simulink model "Experiment_1_cs"  (R2022b)
settings: Solver=ode5  StartTime=0.0  StopTime=30  FixedStep=1/20  RelTol=1e-3
PreLoadFcn:
  | mbxruntime.callbacks.PreLoadFcn(bdroot);
PostLoadFcn:
  | mbxruntime.callbacks.PostLoadFcn(bdroot);
InitFcn:
  | mbxruntime.callbacks.InitFcn(bdroot);
StartFcn:
  | mbxruntime.callbacks.StartFcn(bdroot);
StopFcn:
  | mbxruntime.callbacks.StopFcn(bdroot);
model workspace (MAT data in the model file):
  mbox_table : object (value not decoded)
  model_closed = 0
  sim_status = 0
undefined symbols (not defined in the file or in its folder): blockPath, DiscIntNeverNeededParam, warningInitialVelocity, x0
libraries: PreScanSimulinkLibrary x32, simulink x23, simulink_extras x10
(part 7 of 8)

== system Experiment_1_cs/Male_Old_White_WithStick_1/Trajectories/Traj2State1/Traj2State2/Traj2MuxState_Ext/demux ==
  traj : Inport
  Demux : Demux  Outputs=18
  x : Outport
  y : Outport  Port=2
  z : Outport  Port=3
  velx : Outport  Port=4
  vely : Outport  Port=5
  velz : Outport  Port=6
  R : Outport  Port=7
  P : Outport  Port=8
  Y : Outport  Port=9
  velR : Outport  Port=10
  velP : Outport  Port=11
  velY : Outport  Port=12
  accx : Outport  Port=13
  accy : Outport  Port=14
  accz : Outport  Port=15
  accR : Outport  Port=16
  accP : Outport  Port=17
  accY : Outport  Port=18
  wires:
  Demux/18 -> accY/1
  Demux/17 -> accP/1
  Demux/16 -> accR/1
  Demux/15 -> accz/1
  Demux/14 -> accy/1
  Demux/13 -> accx/1
  Demux/12 -> velY/1
  Demux/11 -> velP/1
  Demux/10 -> velR/1
  Demux/9 -> velz/1
  Demux/8 -> vely/1
  Demux/7 -> velx/1
  Demux/6 -> Y/1
  Demux/5 -> P/1
  traj/1 -> Demux/1
  Demux/4 -> R/1
  Demux/3 -> z/1
  Demux/2 -> y/1
  Demux/1 -> x/1

== system Experiment_1_cs/Man_200_1/Trajectories/Traj2State1/Traj2State2/Traj2MuxState_Ext/demux ==
  traj : Inport
  Demux : Demux  Outputs=18
  x : Outport
  y : Outport  Port=2
  z : Outport  Port=3
  velx : Outport  Port=4
  vely : Outport  Port=5
  velz : Outport  Port=6
  R : Outport  Port=7
  P : Outport  Port=8
  Y : Outport  Port=9
  velR : Outport  Port=10
  velP : Outport  Port=11
  velY : Outport  Port=12
  accx : Outport  Port=13
  accy : Outport  Port=14
  accz : Outport  Port=15
  accR : Outport  Port=16
  accP : Outport  Port=17
  accY : Outport  Port=18
  wires:
  Demux/18 -> accY/1
  Demux/17 -> accP/1
  Demux/16 -> accR/1
  Demux/15 -> accz/1
  Demux/14 -> accy/1
  Demux/13 -> accx/1
  Demux/12 -> velY/1
  Demux/11 -> velP/1
  Demux/10 -> velR/1
  Demux/9 -> velz/1
  Demux/8 -> vely/1
  Demux/7 -> velx/1
  Demux/6 -> Y/1
  Demux/5 -> P/1
  traj/1 -> Demux/1
  Demux/4 -> R/1
  Demux/3 -> z/1
  Demux/2 -> y/1
  Demux/1 -> x/1

== system Experiment_1_cs/Nissan_Cabstar_Boxtruck_1/Trajectories/Traj2State1/Traj2State2/Traj2MuxState_Ext/demux ==
  traj : Inport
  Demux : Demux  Outputs=18
  x : Outport
  y : Outport  Port=2
  z : Outport  Port=3
  velx : Outport  Port=4
  vely : Outport  Port=5
  velz : Outport  Port=6
  R : Outport  Port=7
  P : Outport  Port=8
  Y : Outport  Port=9
  velR : Outport  Port=10
  velP : Outport  Port=11
  velY : Outport  Port=12
  accx : Outport  Port=13
  accy : Outport  Port=14
  accz : Outport  Port=15
  accR : Outport  Port=16
  accP : Outport  Port=17
  accY : Outport  Port=18
  wires:
  Demux/18 -> accY/1
  Demux/17 -> accP/1
  Demux/16 -> accR/1
  Demux/15 -> accz/1
  Demux/14 -> accy/1
  Demux/13 -> accx/1
  Demux/12 -> velY/1
  Demux/11 -> velP/1
  Demux/10 -> velR/1
  Demux/9 -> velz/1
  Demux/8 -> vely/1
  Demux/7 -> velx/1
  Demux/6 -> Y/1
  Demux/5 -> P/1
  traj/1 -> Demux/1
  Demux/4 -> R/1
  Demux/3 -> z/1
  Demux/2 -> y/1
  Demux/1 -> x/1

== system Experiment_1_cs/Audi_A8_Sedan_1/Dynamics_Simple/Chassis/Bicycle_model_[XYZ]/X_Motion/Max RPM and zero- velocity detection/Configurable Subsystem ==
  Step : Step  Time=0.0001  Before=1  After=0  SampleTime=0
  Out1 : Outport
  wires:
  Step/1 -> Out1/1

== system Experiment_1_cs/Audi_A8_Sedan_1/Dynamics_Simple/Chassis/Bicycle_model_[XYZ]/X_Motion/Max RPM and zero- velocity detection/SR-Memory ==
  Signal : Inport
  Set : Inport  Port=2
  Reset : Inport  Port=3
  Constant : Constant  Value=0
  Detect Rise Positive : simulink/Logic and Bit Operations/Detect Rise Positive  vinit=0  OutDataTypeStr=uint8
  Detect Rise Positive1 : simulink/Logic and Bit Operations/Detect Rise Positive  vinit=0  OutDataTypeStr=uint8
  Manual Switch : ManualSwitch
  Manual Switch1 : ManualSwitch
  Switch : Switch  Criteria=u2 ~= 0  SaturateOnIntegerOverflow=off  InputSameDT=off
  Switch1 : Switch  Criteria=u2 ~= 0  SaturateOnIntegerOverflow=off  InputSameDT=off
  Unit Delay : UnitDelay  SampleTime=-1  HasFrameUpgradeWarning=on
  Out : Outport
  wires:
  Constant/1 -> Switch1/1
  Switch/1 -> Switch1/3
  Switch1/1 -> Unit Delay/1, Out/1
  Manual Switch1/1 -> Switch1/2
  Reset/1 -> Manual Switch1/2, Detect Rise Positive1/1
  Detect Rise Positive1/1 -> Manual Switch1/1
  Signal/1 -> Switch/1
  Unit Delay/1 -> Switch/3
  Set/1 -> Detect Rise Positive/1, Manual Switch/2
  Detect Rise Positive/1 -> Manual Switch/1
  Manual Switch/1 -> Switch/2

== matlab function Experiment_1_cs/Audi_A8_Sedan_1/perception module/MATLAB Function2 ==
  data: obs_x input; obs_y input; obs_v input; obs_heading input; obs_id input
function plot_obstacles_vcs(obs_x, obs_y, obs_v, obs_heading, obs_id)
% Simulink-friendly Visualization Function

% 声明绘图函数为 extrinsic
coder.extrinsic('figure','clf','hold','grid','axis','xlim','ylim','xlabel','ylabel','title');
coder.extrinsic('plot','quiver','text','fill','legend');
coder.extrinsic('sprintf');

persistent figCreated;

% 初始化图
if isempty(figCreated)
    figure(100);
    figCreated = true;
end

figure(100);
clf; hold on; grid on; axis equal;

% 坐标范围
xlim([-20 80]);
ylim([-50 50]);
xlabel('X_{VCS} (m)');
ylabel('Y_{VCS} (m)');
title('Obstacle Positions in VCS');

%% ======================
%       主车矩形
% ======================
Lh = 5;   % 主车长
Wh = 2;   % 主车宽
hd = 0;   % 主车朝向始终沿 +X

% 主车矩形点
rect_host = [
    Lh/2,  Wh/2;
    Lh/2, -Wh/2;
   -Lh/2, -Wh/2;
   -Lh/2,  Wh/2
];

% 主车旋转矩阵
R = [cos(hd) -sin(hd); sin(hd) cos(hd)];
rect_host_rot = (R * rect_host')';
rect_host_final = rect_host_rot + [0, 0];

% 绘制主车矩形（蓝色）
fill(rect_host_final(:,1), rect_host_final(:,2), ...
    [0.2 0.6 1.0], 'FaceAlpha',0.4, 'EdgeColor','b', 'LineWidth',2);

text(0, -1.5, 'Host Car', 'Color','b','FontSize',12,'FontWeight','bold');

%% ======================
%       障碍物绘制
% ======================
for i = 1:length(obs_x)
    if isnan(obs_x(i)), continue; end

    ox = obs_x(i);
    oy = obs_y(i);
    v  = obs_v(i);
    hd = obs_heading(i);
    oid = obs_id(i);

    % 速度箭头
    quiver(ox, oy, v*cos(hd), v*sin(hd), 0.5, 'b', 'LineWidth', 1.5);

    %% ========== 障碍车辆 (ID == 42/54) ==========
    if oid == 42 || oid == 54
        L = 5; W = 2;

        rect = [
            L/2,  W/2;
            L/2, -W/2;
           -L/2, -W/2;
           -L/2,  W/2
        ];

        R = [cos(hd) -sin(hd); sin(hd) cos(hd)];
        rect_rot = (R * rect')';
        rect_final = rect_rot + [ox, oy];

        fill(rect_final(:,1), rect_final(:,2), [0.3 0.8 0.3], ...
            'FaceAlpha',0.4, 'EdgeColor','g', 'LineWidth',2);

        text(ox, oy, 'Car(42)', 'Color','g','FontSize',12,'FontWeight','bold');

    else
        %% 普通障碍物
        plot(ox, oy, 'ro', 'MarkerFaceColor', 'r');
        text(ox + 0.3, oy + 0.3, sprintf('%d', int32(oid)), ...
            'Color','y','FontSize',12,'FontWeight','bold');
    end
end

legend('Velocity','Host');

end

== matlab function Experiment_1_cs/Cloud Computing Systerm/Dangerous Check/MATLAB Function ==
  settings: updateMethod=DISCRETE
  data: no_signal_zone_x input; ego_y input; lane0_y input; target_y output; lane1_y input; lane2_y input; last_target_y input; obs_x_set_gcs input; obs_y_set_gcs input; obs_v_set_gcs input; obs_heading_set_gcs input; obs_ID_set input; ego_x input; ego_v input; ego_heading input; ego_yawrate input; last_target_v input; target_v output; time input; out_state output; has_signal output; danger_level output; action output; collision_info output Bus: collision_info_bus
function [target_y, target_v, out_state, has_signal, danger_level, action, collision_info] = ...
    fcn(no_signal_zone_x, ego_y, lane0_y, lane1_y, lane2_y, last_target_y, ...
        obs_x_set_gcs, obs_y_set_gcs, obs_v_set_gcs, obs_heading_set_gcs, ...
        obs_ID_set, ego_x, ego_v, ego_heading, ego_yawrate, last_target_v, time)


%% ------------------------------------------------------
% Persistent Variables
%% ------------------------------------------------------
persistent first_run stored_target_y stored_target_v state block_until_time
action = 0;
collision_info.obs_id = int32(-1);
collision_info.time = -1;

if isempty(first_run)
    first_run = true;
    stored_target_y = 0;
    stored_target_v = 0;
    state = 0;
    block_until_time = 0;
end

%% Parameters
dt = 0.05;
recommond_speed = 15;
lane_width = 3.5;
max_acc = 2;
max_de_acc = -3.5;

ego_heading = wrapToPi(-deg2rad(ego_heading - 90));
lane_y_all = [lane0_y, lane1_y, lane2_y];

%% Signal availability
has_signal = (ego_x < no_signal_zone_x);

%% =============== CASE 1: LOST SIGNAL ===================
if ~has_signal
    stored_target_v = 0;
    stored_target_y = 0;
    state = 0;

    % Danger level 依旧保留
    danger_level = calc_lost_signal_danger( ...
        ego_x, ego_y, ego_heading, ...
        obs_x_set_gcs, obs_y_set_gcs, obs_v_set_gcs, obs_heading_set_gcs, ...
        obs_ID_set, lane_y_all, lane_width);

    % ⭐ 新增：调用 analyze_danger
    [danger_ns, tx_ns] = analyze_danger( ...
        ego_x, ego_y, ego_v, ego_heading, ...
        obs_x_set_gcs, obs_y_set_gcs, obs_v_set_gcs, ...
        obs_heading_set_gcs, obs_ID_set, lane_y_all, lane_width);

    % 找最危险 lane（TTC 最小）
    ttc_list = tx_ns(:,1);
    [min_ttc, idx_lane] = min(ttc_list);

    if min_ttc < 99
        collision_info.obs_id = int32(danger_ns(idx_lane,2));
        collision_info.time   = min_ttc;
    else
        collision_info.obs_id = int32(-1);
        collision_info.time   = 999;
    end

    % 输出保持
    target_v = stored_target_v;
    target_y = stored_target_y;
    out_state = state;
    action = 0;
    return;
end

%% =============== FIRST RUN ===================
if first_run
    [~, idx_lane] = min(abs(ego_y - lane_y_all));
    stored_target_y = lane_y_all(idx_lane);
    stored_target_v = recommond_speed;

    first_run = false;

    target_y = stored_target_y;
    target_v = stored_target_v;
    out_state = state;
    danger_level = 0;
    action = 0;
    return;
end

%% =============== NORMAL MODE ===================
stored_target_y = last_target_y;
stored_target_v = last_target_v;

%% Danger Analysis
[danger, tx_lane] = analyze_danger( ...
    ego_x, ego_y, ego_v, ego_heading, ...
    obs_x_set_gcs, obs_y_set_gcs, obs_v_set_gcs, obs_heading_set_gcs, obs_ID_set, ...
    lane_y_all, lane_width);

% Determine lane index (scalar)
lane_idx = 1;
min_val = abs(stored_target_y - lane_y_all(1));
for ii = 2:3
    if abs(stored_target_y - lane_y_all(ii)) < min_val
        min_val = abs(stored_target_y - lane_y_all(ii));
        lane_idx = ii;
    end
end

is_danger = danger(lane_idx, 1);
t_lane  = tx_lane(lane_idx, 1);
x_lane  = tx_lane(lane_idx, 2);
if is_danger
    collision_info.obs_id = int32(danger(lane_idx, 2));
    collision_info.time = t_lane;
end

%% --------------------- State Machine ---------------------
switch state

case 0   % KEEP
    action = 0;
    block_until_time = time;

    if is_danger
        state = 1;
    else
        stored_target_v = min(stored_target_v + max_acc*dt, recommond_speed);
    end

case 1   % BRAKE
    if is_danger
        d_brake = ego_v^2 / (2*abs(max_de_acc));
        dx_conflict = x_lane - ego_x;

        if d_brake < dx_conflict - 6
            stored_target_v = last_target_v + max_de_acc * dt;
            action = 2;

            obs_id = danger(lane_idx,2);
            idx_obs = find(obs_ID_set == obs_id, 1);
            if isempty(idx_obs), idx_obs = 1; end

            vy = obs_v_set_gcs(idx_obs) * sin(obs_heading_set_gcs(idx_obs));

            block_until_time = time + min(t_lane, (lane_width/2)/max(abs(vy),0.01));

        else
            % change lane
            
            if lane_idx == 1
                cand = 2;
            elseif lane_idx == 3
                cand = 2;
            else
                cand = [1, 3];
            end
        
            % 从候选车道里找一个安全车道
            new_lane = lane_idx; % 默认保持
            for ci = 1:length(cand)
                if ~danger(cand(ci),1)
                    new_lane = cand(ci);
                    break;
                end
            end

            stored_target_y = lane_y_all(new_lane);
            state = 2;
            action = 3;
        end

        % failsafe: too slow but still dangerous
        obs_id = danger(lane_idx, 2);
        obs_v_risk = 999;
        % 手写一个确定的标量查找
        for ii = 1:length(obs_ID_set)
            if obs_ID_set(ii) == obs_id
                obs_v_risk = obs_v_set_gcs(ii);
                break;
            end
        end
        if (ego_v < 5 || obs_v_risk < 0.2)&& is_danger
            new_lane = lane_idx;
            found = false;

            for li = 1:3
                if danger(li,1)==false
                    new_lane = li;
                    found = true;
                    break;
                end
            end

            if ~found
                action = 4;
            else
                stored_target_y = lane_y_all(new_lane);
                state = 2;
            end
        end

    else
        state = 3;
        action = 1;
    end

case 2   % CHANGE LANE
    block_until_time = time + 0.5;
    stored_target_v = last_target_v;
    state = 3;
    action = 3;

case 3   % BLOCK
    if time >= block_until_time
        state = 0;
    end
    stored_target_v = last_target_v;
    action = 1;

end

%% Outputs
target_y = stored_target_y;
target_v = stored_target_v;
out_state = state;
danger_level = 0;

end  % END fcn


%% =====================================================================
%%                        analyze_danger
%% =====================================================================
function [danger, tx_lane] = analyze_danger( ...
    ego_x, ego_y, ego_v, ego_heading, ...
    obs_x, obs_y, obs_v, obs_h, obs_ID, lane_y, lane_width)

N = length(obs_ID);

danger = zeros(3,2);           % [is_danger, obs_id]
tx_lane = 99 * ones(3,2);      % [ttc, x_collision]

TIME_THRESHOLD   = 4;

for i = 1:N
    if isnan(obs_ID(i)), continue; end

    %% === 计算真实碰撞点 ===
    [ok, ttc, cx, cy] = ray_intersect(...
        ego_x, ego_y, 0, ego_v, ...
        obs_x(i), obs_y(i), obs_h(i), obs_v(i));

    % 不发生碰撞
    if ~ok, continue; end

    % 碰撞时间过长 → 不危险
    if ttc > TIME_THRESHOLD + 1
        continue;
    end


    %% === 判断碰撞点属于哪个 lane ===
    for j = 1:3

        if abs(cy - lane_y(j)) < lane_width/2

            danger(j,1) = 1;            % 标记危险
            danger(j,2) = obs_ID(i);    % 责任障碍物
            tx_lane(j,1) = ttc;         % 真实 TTC
            tx_lane(j,2) = cx;          % 碰撞 X 坐标
        end
    end
end

end





%% =====================================================================
%%                     calc_lost_signal_danger
%% =====================================================================
function danger_level = calc_lost_signal_danger(ego_x, ego_y, ego_heading, ...
    obs_x, obs_y, obs_v, obs_h, obs_ID, lane_y_all, lane_width)

danger_level = 0;

N = length(obs_ID);
if N == 0
    return;
end

% Find nearest lane
lane_idx = 1;
min_dist = abs(ego_y - lane_y_all(1));
for j = 2:3
    if abs(ego_y - lane_y_all(j)) < min_dist
        min_dist = abs(ego_y - lane_y_all(j));
        lane_idx = j;
    end
end

t_min = 1e9;  % scalar

for k = 1:N
    if isnan(obs_ID(k))
        continue;
    end

    vy = obs_v(k) * sin(obs_h(k));
    vx = obs_v(k) * cos(obs_h(k));

    % ----- Compute t_lane -----
    if abs(obs_y(k) - lane_y_all(lane_idx)) < lane_width/2
        t_lane = 0;

    elseif abs(vy) < 0.01
        continue;

    else
        t_lane = (lane_y_all(lane_idx) - obs_y(k)) / vy;
        if t_lane <= 0
            continue;
        end
    end

    if t_lane < t_min
        t_min = t_lane;
    end
end

% ----- Level mapping -----
if t_min < 3
    danger_level = 3;
elseif t_min < 5
    danger_level = 2;
elseif t_min < 10
    danger_level = 1;
end

end


%% =====================================================================
%%                       ray_intersect
%% =====================================================================
function [is_possible, collision_time, collision_x, collision_y] = ...
    ray_intersect(x1,y1,h1,v1, x2,y2,h2,v2)

% 默认返回
is_possible = false;
collision_time = Inf;
collision_x = NaN;
collision_y = NaN;

% Heading unit vectors
H1 = [cos(h1), sin(h1)];
H2 = [cos(h2), sin(h2)];

% If any vehicle is stationary, still OK
V1 = v1*H1;
V2 = v2*H2;

% Relative position
rx = x2 - x1;
ry = y2 - y1;

% Relative velocity
vx_rel = V2(1) - V1(1);
vy_rel = V2(2) - V1(2);

% Solve linear system:
% x1 + V1*t = x2 + V2*t2  → (V1 - V2)*t = r
A = [V1(1)-V2(1), -(V1(1)-V2(1));
     V1(2)-V2(2), -(V1(2)-V2(2))];

% But easier: directly solve t1, t2 for ray intersection:
den = H1(1)*H2(2) - H1(2)*H2(1);
if abs(den) < 1e-9
    return; % almost parallel
end

t1 = ( rx*H2(2) - ry*H2(1) ) / den; % ego
t2 = ( rx*H1(2) - ry*H1(1) ) / den; % obs

% Must be forward time
if t1 < 0 || t2 < 0
    if abs(y2 -y1) < 2
        collision_y = y1;
        collision_x = x1 + H1(1)*t1;
        collision_time = (collision_x - x1) / v1;
        is_possible = true;
    end
    return;
end

% Convert param t1 to real physical time
% param_t1 is distance along ray direction, so:
if v1 < 0.01
    return;
end

collision_time = t1 / v1;

% Compute collision point
collision_x = x1 + H1(1)*t1;
collision_y = y1 + H1(2)*t1;

% Mark valid
is_possible = true;
end

== matlab function Experiment_1_cs/Audi_A8_Sedan_1/perception module/MATLAB Function ==
  data: host_x input; obs_x_set_gcs output; host_y input; host_heading_xy input; obs_range input; obs_theta input; obs_velocity input; obs_velocity_heading input; obs_y_set_gcs output; obs_velocity_set_gcs output; obs_heading_set_gcs output; obs_ID_set output; obs_ID input
function [obs_x_set_gcs,obs_y_set_gcs,obs_velocity_set_gcs,obs_heading_set_gcs, obs_ID_set] = ...
    fcn(host_x, host_y, host_heading_xy, obs_range, obs_theta, obs_velocity, obs_velocity_heading, obs_ID)
%gcs 全局坐标系global coordinate system
%该函数是感知模块，输出障碍物的位置，速度大小，速度方向与世界坐标系x轴的夹角
%输入：定位信息host_x,host_y,host_heading_xy 世界坐标系
%      障碍物在传感器坐标系下的极坐标range，theta
%      障碍物的速度大小 velocity
%      障碍物的速度方向与x轴的夹角 heading
%输出：障碍物在世界坐标系下的坐标 x y v v与x轴的夹角heading
%      注意输出的heading是障碍物的速度heading，不是障碍物的几何heading

%传感器最多输出10个障碍物信息，但是事先不知道有多少个障碍物，所以要做个缓冲

%输出初始化
obs_x_set_gcs = ones(10,1)*nan;
obs_y_set_gcs = ones(10,1)*nan;
obs_velocity_set_gcs = ones(10,1)*nan;
obs_heading_set_gcs = ones(10,1)*nan;
obs_ID_set = ones(10, 1) * nan;
host_heading_xy = deg2rad(-host_heading_xy + 90);
%传感器极坐标的角度顺时针为正，世界坐标是逆时针为正
theta_transfer = -obs_theta* pi / 180;
%velocity的方向以北为0度，世界坐标是以东为0度。
heading_transfer = (-obs_velocity_heading + 90*ones(10,1)) * pi / 180;
%计算障碍物到传感器的x方向距离，y 方向距离
x_transfer = obs_range.* cos(theta_transfer + host_heading_xy);
y_transfer = obs_range.* sin(theta_transfer + host_heading_xy);

%计算障碍物的世界坐标
for i = 1:length(obs_range)
    if obs_range(i) ~= 0
        obs_x_set_gcs(i) = x_transfer(i) + host_x + 2.16*cos(host_heading_xy);
        obs_y_set_gcs(i) = y_transfer(i) + host_y + 2.16*sin(host_heading_xy);
        obs_heading_set_gcs(i) = wrapToPi(heading_transfer(i));
        obs_velocity_set_gcs(i) = obs_velocity(i);
        obs_ID_set(i) = obs_ID(i);
    end
end

== matlab function Experiment_1_cs/Audi_A8_Sedan_1/perception module/MATLAB Function3 ==
  data: host_x input; host_y input; host_heading_xy input; x_in input; x_out output; y_in input; v_in input; h_in input; id_in input; y_out output; v_out output; h_out output; id_out output
function [x_out, y_out, v_out, h_out, id_out] = ...
    filter_occlusion_gcs(host_x, host_y, host_heading_xy, ...
                         x_in, y_in, v_in, h_in, id_in)
% 全局坐标系 (GCS) 遮挡过滤
% 输入/输出均为 10×1，兼容 Simulink
% 遮挡规则：
%    - 按主车 → 障碍物的方位角排序（bearing）
%    - 相邻角度差 < 阈值 → 认为可能遮挡
%    - 距离较远者被遮挡

coder.extrinsic('disp');
coder.extrinsic('sprintf');

host_heading_xy = deg2rad(-host_heading_xy + 90);

% ============================================
% 初始化输出（固定维度 10×1）
% ============================================
x_out  = nan(10,1);
y_out  = nan(10,1);
v_out  = nan(10,1);
h_out  = nan(10,1);
id_out = nan(10,1);

% 过滤有效输入
valid = ~isnan(x_in);
x = x_in(valid);
y = y_in(valid);
v = v_in(valid);
h = h_in(valid);
id = id_in(valid);

if isempty(x)
    return;
end

% ============================================
% 计算 bearing（方位角）和距离
% bearing = 障碍物方向 - 主车朝向
% ============================================

dx = x - host_x;
dy = y - host_y;

bearing = wrapToPi(atan2(dy, dx) - host_heading_xy);
dist    = sqrt(dx.^2 + dy.^2);

% ============================================
% 按 bearing 排序（与 VCS 原理一致）
% ============================================
[bearing_sorted, idx] = sort(bearing);

x = x(idx);
y = y(idx);
v = v(idx);
h = h(idx);
id = id(idx);
dist = dist(idx);

% ============================================
% 遮挡判断
% ============================================
angle_threshold = deg2rad(5);   % 5° 容差
keep = true(size(x));

for i = 1:length(x)
    for j = i+1:length(x)

        % 若角度差超出阈值，后续不需要比较
        if abs(bearing_sorted(j) - bearing_sorted(i)) > angle_threshold
            break;
        end

        % ===== 距离比较：距离远的被遮挡 =====
        if dist(j) > dist(i)
            keep(j) = false;
            msg = sprintf('Obs %d blocks Obs %d', id(i), id(j));
            disp(msg);
        else
            keep(i) = false;
            msg = sprintf('Obs %d blocks Obs %d', id(j), id(i));
            disp(msg);
        end
    end
end

% ============================================
% 保留下未被遮挡的障碍物
% ============================================
x = x(keep);
y = y(keep);
v = v(keep);
h = h(keep);
id = id(keep);

N = length(x);

% ============================================
% 写回输出（固定大小 10×1）
% ============================================
x_out(1:N)  = x;
y_out(1:N)  = y;
v_out(1:N)  = v;
h_out(1:N)  = h;
id_out(1:N) = id;

end

== matlab function Experiment_1_cs/Cloud Computing Systerm/Dangerous Check/MATLAB Function1 ==
  settings: updateMethod=DISCRETE
  data: no_signal_zone_x input; ego_y input; lane0_y input; target_y output; lane1_y input; lane2_y input; last_target_y input; obs_x_set_gcs input; obs_y_set_gcs input; obs_v_set_gcs input; obs_heading_set_gcs input; obs_ID_set input; ego_x input; ego_v input; ego_heading input; ego_yawrate input; last_target_v input; target_v output; time input; out_state output; has_signal output; danger_level output; action output
function [target_y, target_v, out_state, has_signal, danger_level, action] = fcn(no_signal_zone_x, ego_y, lane0_y, lane1_y, lane2_y, last_target_y, obs_x_set_gcs, obs_y_set_gcs, obs_v_set_gcs, ...
    obs_heading_set_gcs, obs_ID_set, ego_x, ego_v, ego_heading, ego_yawrate, last_target_v, time)

persistent first_run stored_target_y stored_target_v over_decc_time block_until_time
% state 0=KEEP, 1=BRAKE, 2=LANE_CHANGE, 3=BLOCK_RECOVER
persistent state avoid_id

ego_heading =-deg2rad(ego_heading-90);
ego_heading = wrapToPi(ego_heading);
recommond_speed = 15;
dt = 0.05;
lane_width = 3.5;
max_de_acc = -2.5;
max_acc = 2;
danger_level = 0;
action = 0; %  0: 正常行驶 1: 保持状态 2：发现危险，降速避让中 3： 发现危险，变道避让中


has_signal = ego_x < no_signal_zone_x;




if has_signal

    % =========================
    % 初始化 persistent
    % =========================
    if isempty(first_run)
        first_run = true;
        stored_target_y = 0;
        stored_target_v = 0;
        state = 0;
        action = 0;
        over_decc_time = -inf;
        block_until_time = -inf;
    end



    if first_run
        % ================
        % 第一次运行：找最近车道
        % ================
        danger_level = 0;

        d0 = abs(ego_y - lane0_y);
        d1 = abs(ego_y - lane1_y);
        d2 = abs(ego_y - lane2_y);

        [~, idx] = min([d0, d1, d2]);

        if idx == 1
            stored_target_y = lane0_y;
        elseif idx == 2
            stored_target_y = lane1_y;
        else
            stored_target_y = lane2_y;
        end
        stored_target_v = recommond_speed;

        first_run = false;     % 从下一周期开始锁定目标车道

    else
        % ================
        % 后续周期：默认保持上一周期车道，检查有无碰撞风险
        % ================
        stored_target_y = last_target_y;
        stored_target_v = last_target_v;
        % 障碍物预测，计算每个障碍物到达三个车道的时间t, 和x, 然后看t s过后自车所在的x
        valid_idx = ~isnan(obs_ID_set);
        N = sum(valid_idx);
        if N == 0
            % 没有要处理的障碍物， no obs
            state = 0;
            target_y = last_target_y;
            target_v = min(last_target_v + max_acc * dt, recommond_speed);
            out_state = 0;
            action = 0;
            danger_level = 0;
            return
        end
        % 三条道路是否有危险, (是否危险，造成危险的障碍物ID)
        danger = zeros(3,2);
        lane_y = [lane0_y, lane1_y, lane2_y];
        % 记录障碍物到达每个时间和x
        lane_width = 3.5;

        tx_lane = 99 * ones(3,2);

        valid_idx = find(~isnan(obs_ID_set));
        N = length(valid_idx);

        for ii = 1:N
            i = valid_idx(ii);


            obs_y = obs_y_set_gcs(i);
            obs_x = obs_x_set_gcs(i);
            obs_v = obs_v_set_gcs(i);
            obs_h = obs_heading_set_gcs(i);

            obs_vy = obs_v * sin(obs_h);
            obs_vx = obs_v * cos(obs_h);

            risk_flag = ray_intersect(ego_x, stored_target_y, 0, obs_x, obs_y, obs_h);


            if ~risk_flag
                continue;
            end

            for j = 1:3

                % ===================
                % 情况 1：障碍物就在此车道 → 立即评估
                % ===================
                if abs(obs_y - lane_y(j)) < lane_width/2
                    t_lane = 0;

                    % ===================
                    % 情况 2：不在车道，且 vy≈0 → 永远不会到此车道
                    % ===================
                elseif abs(obs_vy) < 0.01
                    t_lane = inf;

                    % ===================
                    % 情况 3：正常横向速度 → 可计算到达时间
                    % ===================
                else
                    t_lane = (lane_y(j) - obs_y) / obs_vy;
                    if t_lane <= 0
                        t_lane = inf;  % 朝反方向运动，不会到达
                    end
                end

                % 跳过无效时间
                if isinf(t_lane)
                    continue;
                end

                % 障碍物到达 j 车道中心线时的 x
                x_lane = obs_x + obs_vx * t_lane;

                % 自车未来 x
                ego_x_tlane = ego_x + ego_v * t_lane * cos(ego_heading);

                % 若纵向差小于阈值 → 此车道危险
                if  (t_lane < 4 && t_lane >= 0) || abs(ego_x_tlane - x_lane) < max(10, 2 * ego_v) || (t_lane < 0.1 && abs(ego_x - obs_x) < 20 && abs(ego_y - obs_y) < 2.5)
                    danger(j, 1) = true;
                    danger(j, 2) = obs_ID_set(i);
                    tx_lane(j,1) = t_lane;
                    tx_lane(j,2) = x_lane;
                end
            end
        end

        if stored_target_y == lane0_y
            is_danger = danger(1,1);
            switch state
                case 0
                    block_until_time = 0;
                    action = 0;
                    if is_danger
                        state = 1;
                    else
                        % 不危险，正常加速
                        stored_target_v =  min(stored_target_v + max_acc * dt, recommond_speed);
                        stored_target_y = stored_target_y;
                    end
                case 1
                    if is_danger
                        % 能否通过刹车避免
                        d_brake = ego_v^2/(2*abs(max_de_acc));
                        dx_conflict = tx_lane(1,2) - ego_x;
                        if d_brake < dx_conflict - 6
                            action = 2;
                            % 继续减速
                            stored_target_v = last_target_v + max_de_acc * dt;
                            stored_target_y = last_target_y;
                            obs_id = danger(1, 2);
                            idx = find(obs_ID_set == obs_id, 1);
                            obs_v  = obs_v_set_gcs(idx);
                            obs_h  = obs_heading_set_gcs(idx);
                            obs_vy = obs_v * sin(obs_h);
                            block_until_time = time + tx_lane(1, 1) + (lane_width/2)/(abs(obs_vy)) + 0.5;
                        else
                            % 不能刹住，得变道
                            if ~danger(2, 1)
                                action = 3;
                                stored_target_y = lane1_y;
                                stored_target_v = last_target_v;
                                state = 2;
                            end
                        end
                    else
                        % 危险解除，进入保持阶段
                        state = 3;
                        action = 1;
                    end
                case 2
                    % 变道状态
                    % 刚变道的那一下，不允许加速
                    block_until_time = time + 0.5;
                    stored_target_v = last_target_v;
                    stored_target_y = last_target_y;
                    state = 3;
                    action = 3;
                case 3
                    if time >= block_until_time
                        state = 0;
                    end
                    % 不管是变道还是刹车，路径和速度都和传进来的一样
                    stored_target_v = last_target_v;
                    stored_target_y = last_target_y;
                    action = 1;
            end
        elseif stored_target_y == lane1_y
            is_danger = danger(2,1);
            switch state
                case 0
                    action = 0;
                    block_until_time = 0;
                    if is_danger
                        state = 1;
                    else
                        % 不危险，正常加速
                        stored_target_v =  min(last_target_v + max_acc * dt, recommond_speed);
                        stored_target_y = stored_target_y;
                    end
                case 1
                    if is_danger
                        % 能否通过刹车避免
                        d_brake = ego_v^2/(2*abs(max_de_acc));
                        dx_conflict = tx_lane(2,2) - ego_x;
                        if d_brake < dx_conflict - 6 % buffer
                            % 继续减速
                            stored_target_v = last_target_v + max_de_acc * dt;
                            stored_target_y = last_target_y;
                            obs_id = danger(2, 2);
                            idx = find(obs_ID_set == obs_id, 1);
                            obs_v  = obs_v_set_gcs(idx);
                            obs_h  = obs_heading_set_gcs(idx);
                            obs_vy = obs_v * sin(obs_h);
                            block_until_time = time + tx_lane(2, 1) + (lane_width/2)/(abs(obs_vy)) + 0.5;
                            action = 2;
                        else
                            % 不能刹住，得变道
                            if ~danger(1, 1)
                                stored_target_y = lane0_y;
                                stored_target_v = last_target_v;
                                state = 2;
                                action = 3;
                            elseif ~danger(3,1)
                                stored_target_y = lane2_y;
                                stored_target_v = last_target_v;
                                action = 3;
                                state = 2;
                            end
                        end
                    else
                        % 危险解除，进入保持阶段
                        state = 3;
                        action = 1;
                    end
                    if ego_v < 5 && is_danger %都刹到这么小速度了，还有危险，赶紧变道
                        if ~danger(1,1)
                            stored_target_y = lane0_y;
                            state = 2;
                        elseif ~danger(3,1)
                            stored_target_y = lane2_y;
                            state = 2;
                        else
                            action = 4;  % 两边都危险 → 紧急停车
                        end
                    end
                case 2
                    % 变道状态
                    % 刚变道的那一下，不允许加速
                    block_until_time = time + 0.5;
                    stored_target_v = last_target_v;
                    stored_target_y = last_target_y;
                    state = 3;
                    action = 3;
                case 3
                    if time >= block_until_time
                        state = 0;
                    end
                    % 不管是变道还是刹车，路径和速度都和传进来的一样
                    stored_target_v = last_target_v;
                    stored_target_y = last_target_y;
                    action = 1;
            end

        elseif stored_target_y == lane2_y
            is_danger = danger(3,1);
            switch state
                case 0
                    action = 0;
                    block_until_time = 0;
                    if is_danger
                        state = 1;
                    else
                        % 不危险，正常加速
                        stored_target_v =  min(stored_target_v + max_acc * dt, recommond_speed);
                        stored_target_y = stored_target_y;
                    end
                case 1
                    if is_danger
                        % 能否通过刹车避免
                        d_brake = ego_v^2/(2*abs(max_de_acc));
                        dx_conflict = tx_lane(3,2) - ego_x;
                        if d_brake < dx_conflict - 6
                            % 继续减速
                            stored_target_v = last_target_v + max_de_acc * dt;
                            stored_target_y = last_target_y;
                            obs_id = danger(3, 2);
                            idx = find(obs_ID_set == obs_id, 1);
                            obs_v  = obs_v_set_gcs(idx);
                            obs_h  = obs_heading_set_gcs(idx);
                            obs_vy = obs_v * sin(obs_h);
                            block_until_time = time + tx_lane(3, 1) + (lane_width/2)/(abs(obs_vy)) + 0.5;
                            action = 2;
                        else
                            % 不能刹住，得变道
                            if ~danger(1, 1)
                                stored_target_y = lane1_y;
                                stored_target_v = last_target_v;
                                state = 2;
                                action = 3;
                            end
                        end
                    else
                        % 危险解除，进入保持阶段
                        state = 3;
                        action = 1;
                    end
                case 2
                    % 变道状态
                    % 刚变道的那一下，不允许加速
                    block_until_time = time + 0.5;
                    stored_target_v = last_target_v;
                    stored_target_y = last_target_y;
                    state = 3;
                    action = 3;
                case 3
                    if time >= block_until_time
                        state = 0;
                    end
                    % 不管是变道还是刹车，路径和速度都和传进来的一样
                    stored_target_v = last_target_v;
                    stored_target_y = last_target_y;
                    action = 1;
            end
        end

    end
else
    % 没信号区域 只发送提醒信号
    stored_target_v = 0;
    stored_target_y = 0;
    state = 0;
    % 计算危险程度，进行提醒
    % 找到自车所在车道
    d0 = abs(ego_y - lane0_y);
    d1 = abs(ego_y - lane1_y);
    d2 = abs(ego_y - lane2_y);
    [~, idx] = min([d0, d1, d2]);


    % 障碍物预测，计算每个障碍物到达三个车道的时间t, 和x, 然后看t s过后自车所在的x
    valid_idx = ~isnan(obs_ID_set);
    N = sum(valid_idx);
    if N == 0
        % 没有要处理的障碍物， no obs
        target_y = last_target_y;
        target_v = min(last_target_v + max_acc * dt, recommond_speed);
        out_state = 0;
        danger_level = 0;
        return
    end
    % 三条道路是否有危险, (是否危险，造成危险的障碍物ID)
    danger = zeros(3,2);
    lane_y = [lane0_y, lane1_y, lane2_y];
    % 记录障碍物到达每个时间和x
    lane_width = 3.5;

    tx_lane = 99 * ones(3,2);

    valid_idx = find(~isnan(obs_ID_set));
    N = length(valid_idx);

    for ii = 1:N
        i = valid_idx(ii);


        obs_y = obs_y_set_gcs(i);
        obs_x = obs_x_set_gcs(i);
        obs_v = obs_v_set_gcs(i);
        obs_h = obs_heading_set_gcs(i);

        obs_vy = obs_v * sin(obs_h);
        obs_vx = obs_v * cos(obs_h);

        for j = 1:3

            % ===================
            % 情况 1：障碍物就在此车道 → 立即评估
            % ===================
            if abs(obs_y - lane_y(j)) < lane_width/2
                t_lane = 0;

                % ===================
                % 情况 2：不在车道，且 vy≈0 → 永远不会到此车道
                % ===================
            elseif abs(obs_vy) < 0.01
                t_lane = inf;

                % ===================
                % 情况 3：正常横向速度 → 可计算到达时间
                % ===================
            else
                t_lane = (lane_y(j) - obs_y) / obs_vy;
                if t_lane <= 0
                    t_lane = inf;  % 朝反方向运动，不会到达
                end
            end

            % 跳过无效时间
            if isinf(t_lane)
                continue;
            end

            % 障碍物到达 j 车道中心线时的 x
            x_lane = obs_x + obs_vx * t_lane;

            % 自车未来 x
            ego_x_tlane = ego_x + ego_v * t_lane * cos(ego_heading);

            % 若纵向差小于阈值 → 此车道危险
            if abs(ego_x_tlane - x_lane) < 10 || (t_lane < 0.1 && abs(ego_x - obs_x) < 20 && abs(ego_y - obs_y) < 2.5)
                danger(j, 1) = true;
                danger(j, 2) = obs_ID_set(i);
                tx_lane(j,1) = t_lane;
                tx_lane(j,2) = x_lane;
            end
        end
    end

    if danger(idx, 1) == true
        if tx_lane(idx, 1) <= 10 && tx_lane(idx, 1) >= 5
            danger_level = 1;
        elseif tx_lane(idx, 1) < 5 && tx_lane(idx, 1) >= 3
            danger_level = 2;
        elseif tx_lane(idx, 1) < 3 && tx_lane(idx, 1) >= 0
            danger_level = 3;
        else
            danger_level = 0;
        end
    else
        danger_level = 0;
    end

end
% 输出
target_v = stored_target_v;
target_y = stored_target_y;
out_state = state;

end  % function fcn END






%%%%%%%%%%%%%%%%%%%%%%%%%%%%%%%%%%%%%%%%%%%%%%%%%%%%%%%%%%%%%%
%%              Local Function: has_risk
%%%%%%%%%%%%%%%%%%%%%%%%%%%%%%%%%%%%%%%%%%%%%%%%%%%%%%%%%%%%%%
function is_possible = ray_intersect(x1,y1,h1, x2,y2,h2)

% 射线方向
H1 = [cos(h1), sin(h1)];
H2 = [cos(h2), sin(h2)];

% 相对位置
r = [x2-x1, y2-y1];

%===========================
% ① 平行/近平行：直接用最近距离判断
%===========================
diff_rad = abs(wrapToPi(h1 - h2));

if diff_rad < deg2rad(2)
    % ⭐新增：即使平行，也判断最近距离是否过近⭐
    dist_min = abs( r(1)*H1(2) - r(2)*H1(1) );  % r 到 H1 的垂直距离
    is_possible = dist_min < 5;   % 阈值可调
    return;
end

%===========================
% ② 求交点参数
%===========================
den = H1(1)*H2(2) - H1(2)*H2(1);

if abs(den) < 1e-6
    % ⭐新增：平行但不是置信平行 → 最近距离判定⭐
    dist_min = abs( r(1)*H1(2) - r(2)*H1(1) );
    is_possible = dist_min < 5;
    return;
end

t1 = ( r(1)*H2(2) - r(2)*H2(1) ) / den;
t2 = ( r(1)*H1(2) - r(2)*H1(1) ) / den;

%===========================
% ③ 常规：交点必须在射线前方
%===========================
if t1 > 0 && t2 > 0
    is_possible = true;
    return;
end

%===========================
% ④ ⭐新增：交点在后方，但射线靠得很近也应该认为危险 ⭐
%===========================
% 最近点距离
dist_min = abs( r(1)*H1(2) - r(2)*H1(1) );

is_possible = dist_min < 5;   % YOU CAN TUNE THIS

end




%%%%%%%%%%%%%%%%%%%%%%%%%%%%%%%%%%%%%%%%%%%%%%%%%%%%%%%%%%%%%%
%%                       cross2
%%%%%%%%%%%%%%%%%%%%%%%%%%%%%%%%%%%%%%%%%%%%%%%%%%%%%%%%%%%%%%
function c = cross2(a, b)
% a = [ax ay], b = [bx by]
c = a(1)*b(2) - a(2)*b(1);
end


%%%%%%%%%%%%%%%%%%%%%%%%%%%%%%%%%%%%%%%%%%%%%%%%%%%%%%%%%%%%%%
%%                       dot2
%%%%%%%%%%%%%%%%%%%%%%%%%%%%%%%%%%%%%%%%%%%%%%%%%%%%%%%%%%%%%%
function d = dot2(a, b)
% a = [ax ay], b = [bx by]
d = a(1)*b(1) + a(2)*b(2);
end
